simulink model "MX64"  (R2018a)
settings: Solver=VariableStepAuto  StartTime=0.0  StopTime=10.0  MaxStep=2e-04  RelTol=1e-5
values from neighbouring files (symbols this model uses):
  MX106_Te = 1/1000    (= 0.001)    [MX106_init.m]
  MX64_amplifier = MX64_supply_voltage/1024    (= 0.014453125)    [MX64_init.m]
  MX64_inductor = 6.37e-6    (= 6.37e-06)    [MX64_init.m]
  MX64_init_position = 0    [MX64_init.m]
  MX64_Kc = 8e-1    (= 0.8)    [MX64_init.m]
  MX64_Kd = 1/8    (= 0.125)    [MX64_init.m]
  MX64_Ki = 1/1024    (= 0.0009765625)    [MX64_init.m]
  MX64_Kp = 1/8    (= 0.125)    [MX64_init.m]
  MX64_Kv = 9.926e-3    (= 0.009926)    [MX64_init.m]
  MX64_max_speed = 63 * MX64_reduction / 60 * 2 * pi    (= 1319.46891451)    [MX64_init.m]
  MX64_position_gain = 4096 / 2 / pi    (= 651.898646904)    [MX64_init.m]
  MX64_position_offset = pi    (= 3.14159265359)    [MX64_init.m]
  MX64_reduction = 200    [MX64_init.m]
  MX64_stall_current = 5.2    [MX64_init.m]
  MX64_stall_torque = 6.0 / MX64_reduction    (= 0.03)    [MX64_init.m]
  MX64_Te = 1/1000    (= 0.001)    [MX64_init.m]
undefined symbols (not defined in the file or in its folder): MX64_resistor, MX64_speed_gain
libraries: simulink x7, simulink_extras x1
settings Model: Creator=matt  LastModifiedBy=matt

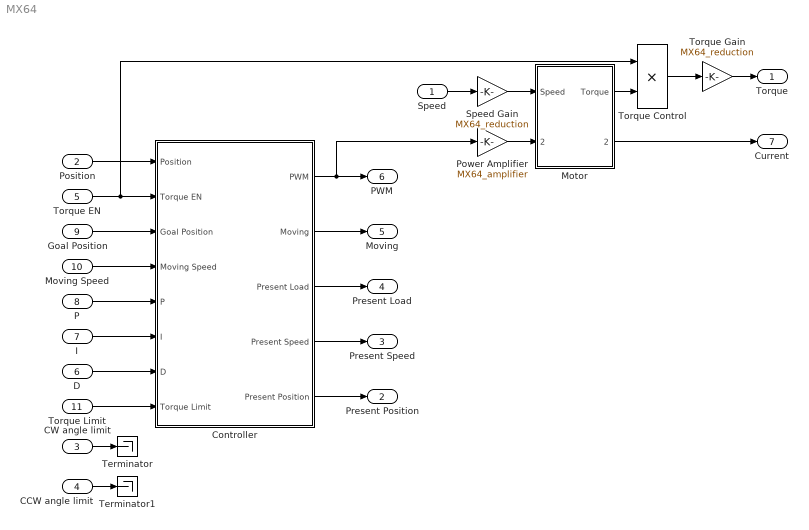
== system MX64 ==
  Speed : Inport
  Position : Inport  Port=2
  CW angle limit : Inport  Port=3  OutDataTypeStr=int16
  CCW angle limit : Inport  Port=4  OutDataTypeStr=int16
  Torque EN : Inport  Port=5  OutDataTypeStr=boolean
  D : Inport  Port=6  OutDataTypeStr=uint8
  I : Inport  Port=7  OutDataTypeStr=uint8
  P : Inport  Port=8  OutDataTypeStr=uint8
  Goal Position : Inport  Port=9
  Moving Speed : Inport  Port=10  OutDataTypeStr=int16
  Torque Limit : Inport  Port=11  OutDataTypeStr=int16
  Controller : Subsystem
  Motor : Subsystem
  Power Amplifier : Gain  Gain=MX64_amplifier  OutDataTypeStr=double
  Speed Gain : Gain  Gain=MX64_reduction
  Terminator : Terminator
  Terminator1 : Terminator
  Torque Control : Product
  Torque Gain : Gain  Gain=MX64_reduction
  Torque : Outport
  Present Position : Outport  Port=2
  Present Speed : Outport  Port=3
  Present Load : Outport  Port=4
  Moving : Outport  Port=5
  PWM : Outport  Port=6
  Current : Outport  Port=7
  wires:
  Controller/5(Present Position) -> Present Position/1
  Controller/3(Present Load) -> Present Load/1
  CW angle limit/1 -> Terminator/1
  Goal Position/1 -> Controller/3(Goal Position)
  Torque Limit/1 -> Controller/8(Torque Limit)
  P/1 -> Controller/5(P)
  Moving Speed/1 -> Controller/4(Moving Speed)
  Torque Control/1 -> Torque Gain/1
  CCW angle limit/1 -> Terminator1/1
  Motor/1(Torque) -> Torque Control/2
  I/1 -> Controller/6(I)
  Torque EN/1 -> Controller/2(Torque EN), Torque Control/1
  Controller/2(Moving) -> Moving/1
  Position/1 -> Controller/1(Position)
  Power Amplifier/1 -> Motor/2(Voltage)
  D/1 -> Controller/7(D)
  Speed/1 -> Speed Gain/1
  Controller/4(Present Speed) -> Present Speed/1
  Controller/1(PWM) -> Power Amplifier/1, PWM/1
  Torque Gain/1 -> Torque/1
  Motor/2(Current) -> Current/1
  Speed Gain/1 -> Motor/1(Speed)

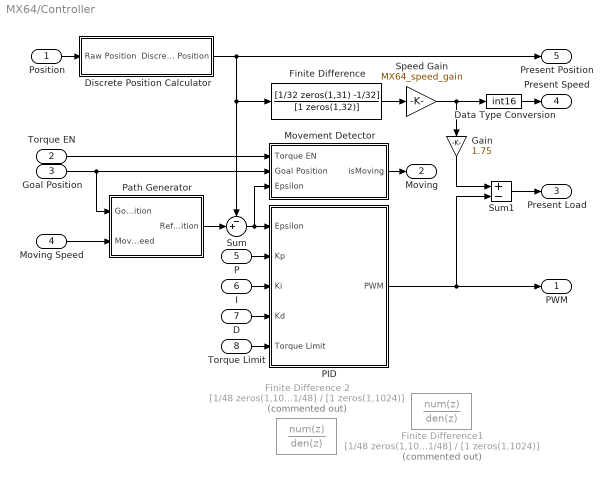
== system MX64/Controller ==
  Position : Inport
  Torque EN : Inport  Port=2
  Goal Position : Inport  Port=3  OutDataTypeStr=int16
  Moving Speed : Inport  Port=4
  P : Inport  Port=5
  I : Inport  Port=6
  D : Inport  Port=7
  Torque Limit : Inport  Port=8
  Data Type Conversion : DataTypeConversion  OutDataTypeStr=int16
  Discrete Position Calculator : Subsystem
  Finite Difference : DiscreteTransferFcn  Numerator=[1/32 zeros(1,31) -1/32]  Denominator=[1 zeros(1,32)]  InitialStates=(MX64_init_position + MX64_position_offset) * MX64_position_gain
  Finite Difference 2 : DiscreteTransferFcn  Commented=on  Numerator=[1/48 zeros(1,1023) -1/48]  Denominator=[1 zeros(1,1024)]  InitialStates=(MX64_init_position + MX64_position_offset) * MX64_position_gain  a0EqualsOne=on
  Finite Difference1 : DiscreteTransferFcn  Commented=on  Numerator=[1/48 zeros(1,1023) -1/48]  Denominator=[1 zeros(1,1024)]  InitialStates=(MX64_init_position + MX64_position_offset) * MX64_position_gain
  Gain : Gain  Gain=1.75  OutDataTypeStr=int16
  Movement Detector : Subsystem
  PID : Subsystem
  Path Generator : Subsystem
  Speed Gain : Gain  Gain=MX64_speed_gain  OutDataTypeStr=double
  Sum : Sum  Inputs=-+|  AccumDataTypeStr=double  OutMin=-4096  OutMax=4096  OutDataTypeStr=double  SaturateOnIntegerOverflow=on
  Sum1 : Sum  Inputs=+-
  PWM : Outport
  Moving : Outport  Port=2
  Present Load : Outport  Port=3
  Present Speed : Outport  Port=4
  Present Position : Outport  Port=5
  wires:
  Movement Detector/1(isMoving) -> Moving/1
  Torque EN/1 -> Movement Detector/1(Torque EN)
  Path Generator/1(Ref Position) -> Sum/2
  Moving Speed/1 -> Path Generator/2(Moving Speed)
  Gain/1 -> Sum1/1
  Sum1/1 -> Present Load/1
  P/1 -> PID/2(Kp)
  I/1 -> PID/3(Ki)
  D/1 -> PID/4(Kd)
  Torque Limit/1 -> PID/5(Torque Limit)
  Data Type Conversion/1 -> Present Speed/1
  Position/1 -> Discrete Position Calculator/1(Raw Position)
  Discrete Position Calculator/1(Discrete Position) -> Finite Difference/1, Sum/1, Present Position/1
  Speed Gain/1 -> Data Type Conversion/1, Gain/1
  PID/1(PWM) -> PWM/1, Sum1/2
  Sum/1 -> PID/1(Epsilon), Movement Detector/3(Epsilon)
  Finite Difference/1 -> Speed Gain/1
  Goal Position/1 -> Path Generator/1(Goal Position), Movement Detector/2(Goal Position)

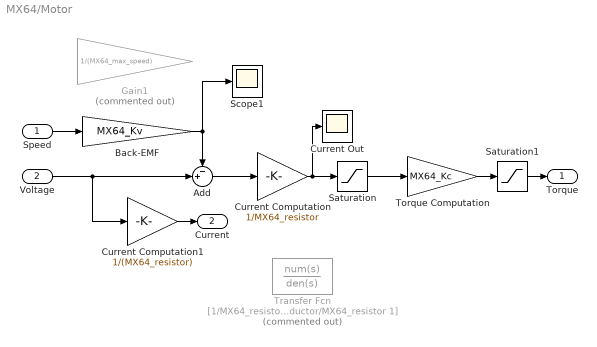
== system MX64/Motor ==
  Speed : Inport
  Voltage : Inport  Port=2
  Add : Sum  Inputs=-+|
  Back-EMF : Gain  Gain=MX64_Kv
  Current Computation : Gain  Gain=1/MX64_resistor
  Current Computation1 : Gain  Gain=1/(MX64_resistor)
  Current Out : Scope
  Gain1 : Gain  Commented=on  Gain=1/(MX64_max_speed)
  Saturation : Saturate  UpperLimit=MX64_stall_current / MX64_reduction  LowerLimit=-MX64_stall_current / MX64_reduction
  Saturation1 : Saturate  UpperLimit=MX64_stall_torque  LowerLimit=-MX64_stall_torque
  Scope1 : Scope
  Torque Computation : Gain  Gain=MX64_Kc
  Transfer Fcn : TransferFcn  Commented=on  Numerator=[1/MX64_resistor]  Denominator=[MX64_inductor/MX64_resistor 1]
  Torque : Outport
  Current : Outport  Port=2
  wires:
  Voltage/1 -> Add/2, Current Computation1/1
  Back-EMF/1 -> Scope1/1, Add/1
  Torque Computation/1 -> Saturation1/1
  Saturation/1 -> Torque Computation/1
  Saturation1/1 -> Torque/1
  Add/1 -> Current Computation/1
  Current Computation1/1 -> Current/1
  Speed/1 -> Back-EMF/1
  Current Computation/1 -> Current Out/1, Saturation/1

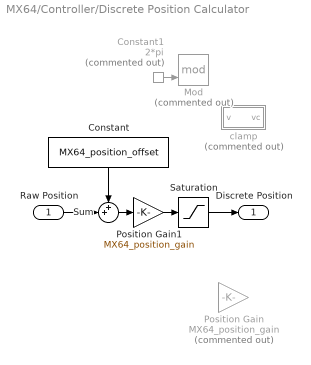
== system MX64/Controller/Discrete Position Calculator ==
  Raw Position : Inport
  Constant : Constant  Value=MX64_position_offset  SampleTime=-1
  Constant1 : Constant  Commented=on  Value=2*pi
  Mod : Math  Commented=on  Operator=mod  SaturateOnIntegerOverflow=on
  Position Gain : Gain  Commented=on  Gain=MX64_position_gain  OutMin=0  OutMax=4095  OutDataTypeStr=int16  SaturateOnIntegerOverflow=on
  Position Gain1 : Gain  Gain=MX64_position_gain  OutMin=0  OutMax=4095  OutDataTypeStr=int16  SampleTime=MX64_Te  SaturateOnIntegerOverflow=on
  Saturation : Saturate  UpperLimit=4095  LowerLimit=0  ZeroCross=off
  Sum : Sum  Inputs=++|
  clamp : Subsystem  Commented=on
  Discrete Position : Outport
  wires:
  Position Gain1/1 -> Saturation/1
  Constant/1 -> Sum/1
  Raw Position/1 -> Sum/2
  Sum/1 -> Position Gain1/1
  ? -> Mod/1
  Constant1/1 -> Mod/2
  Saturation/1 -> Discrete Position/1

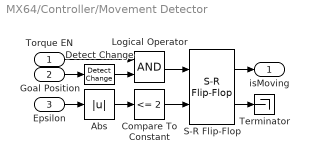
== system MX64/Controller/Movement Detector ==
  Torque EN : Inport
  Goal Position : Inport  Port=2
  Epsilon : Inport  Port=3
  Abs : Abs  ZeroCross=off
  Compare To Constant : simulink/Logic and Bit Operations/Compare To Constant  relop=<=  const=2  OutDataTypeStr=boolean  ZeroCross=off
  Detect Change : simulink/Logic and Bit Operations/Detect Change  vinit=0  OutDataTypeStr=boolean
  Logical Operator : Logic  AllPortsSameDT=off  OutDataTypeStr=boolean
  S-R Flip-Flop : simulink_extras/Flip Flops/S-R Flip-Flop  initial_condition=0
  Terminator : Terminator
  isMoving : Outport
  wires:
  Compare To Constant/1 -> S-R Flip-Flop/2
  Abs/1 -> Compare To Constant/1
  Goal Position/1 -> Detect Change/1
  Detect Change/1 -> Logical Operator/2
  S-R Flip-Flop/2 -> Terminator/1
  Logical Operator/1 -> S-R Flip-Flop/1
  Epsilon/1 -> Abs/1
  S-R Flip-Flop/1 -> isMoving/1
  Torque EN/1 -> Logical Operator/1

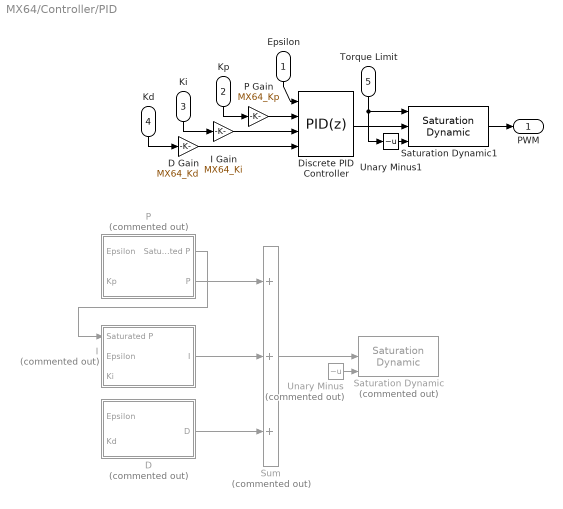
== system MX64/Controller/PID ==
  Epsilon : Inport
  Kp : Inport  Port=2
  Ki : Inport  Port=3
  Kd : Inport  Port=4
  Torque Limit : Inport  Port=5
  D : Subsystem  Commented=on
  D Gain : Gain  Gain=MX64_Kd  OutDataTypeStr=double
  Discrete PID Controller : simulink/Continuous/PID Controller  Controller=PID  TimeDomain=Discrete-time  SampleTime=-1  IntegratorMethod=Forward Euler  FilterMethod=Forward Euler  Form=Parallel  UseFilter=off  ControllerParametersSource=external  P=1  I=1  D=0  N=100  InitialConditionSource=internal  InitialConditionForIntegrator=0  InitialConditionForFilter=0  ExternalReset=none  LimitOutput=off  UpperSaturationLimit=inf  LowerSaturationLimit=-inf  LinearizeAsGain=off  AntiWindupMode=none  Kb=1  TrackingMode=off  Kt=1  PParamMin=[]  PParamMax=[]  IParamMin=[]  IParamMax=[]  DParamMin=[]  DParamMax=[]  NParamMin=[]  NParamMax=[]  KbParamMin=[]  KbParamMax=[]  KtParamMin=[]  KtParamMax=[]  POutMin=[]  POutMax=[]  IOutMin=[]  IOutMax=[]  DOutMin=[]  DOutMax=[]  NOutMin=[]  NOutMax=[]  KbOutMin=[]  KbOutMax=[]  KtOutMin=[]  KtOutMax=[]  IntegratorOutMin=[]  IntegratorOutMax=[]  FilterOutMin=[]  FilterOutMax=[]  SumOutMin=[]  SumOutMax=[]  SumOutDataTypeStr=int16  SumI1OutMin=[]  SumI1OutMax=[]  SumI2OutMin=[]  SumI2OutMax=[]  SumI3OutMin=[]  SumI3OutMax=[]  SumDOutMin=[]  SumDOutMax=[]  SaturationOutMin=[]  SaturationOutMax=[]  IntegratorContinuousStateAttributes=''  IntegratorStateMustResolveToSignalObject=off  IntegratorRTWStateStorageClass=Auto  FilterContinuousStateAttributes=''  FilterStateMustResolveToSignalObject=off  FilterRTWStateStorageClass=Auto  DifferentiatorICPrevScaledInput=0  DifferentiatorOutMin=[]  DifferentiatorOutMax=[]  FilterDiffOutCoefMin=[]  FilterDiffOutCoefMax=[]  SumDenOutMin=[]  SumDenOutMax=[]  SumNumOutMin=[]  SumNumOutMax=[]  ReciprocalOutMin=[]  ReciprocalOutMax=[]  DivideOutMin=[]  DivideOutMax=[]  TunerSelectOption=Transfer Function Based (PID Tuner App)
  I : Subsystem  Commented=on
  I Gain : Gain  Gain=MX64_Ki  OutDataTypeStr=double
  P : Subsystem  Commented=on
  P Gain : Gain  Gain=MX64_Kp  OutDataTypeStr=double
  Saturation Dynamic : simulink/Discontinuities/Saturation Dynamic  Commented=on  OutMin=[]  OutMax=[]  OutDataTypeStr=Inherit: Same as second input  OutDataType=fixdt(1, 16)  OutScaling=2^-10  DoSatur=off
  Saturation Dynamic1 : simulink/Discontinuities/Saturation Dynamic  OutMin=[]  OutMax=[]  OutDataTypeStr=Inherit: Same as second input  OutDataType=fixdt(1, 16)  OutScaling=2^-10  DoSatur=off
  Sum : Sum  Commented=on  Inputs=3  OutDataTypeStr=int16  SaturateOnIntegerOverflow=on
  Unary Minus : UnaryMinus  Commented=on
  Unary Minus1 : UnaryMinus
  PWM : Outport
  wires:
  Unary Minus/1 -> Saturation Dynamic/3
  Sum/1 -> Saturation Dynamic/2
  Epsilon/1 -> Discrete PID Controller/1
  Kp/1 -> P Gain/1
  P/2(P) -> Sum/1
  P/1(Saturated P) -> I/1(Saturated P)
  Ki/1 -> I Gain/1
  I/1(I) -> Sum/2
  D/1(D) -> Sum/3
  P Gain/1 -> Discrete PID Controller/2
  I Gain/1 -> Discrete PID Controller/3
  D Gain/1 -> Discrete PID Controller/4
  Discrete PID Controller/1 -> Saturation Dynamic1/2
  Unary Minus1/1 -> Saturation Dynamic1/3
  Saturation Dynamic1/1 -> PWM/1
  Torque Limit/1 -> Saturation Dynamic1/1, Unary Minus1/1
  Kd/1 -> D Gain/1

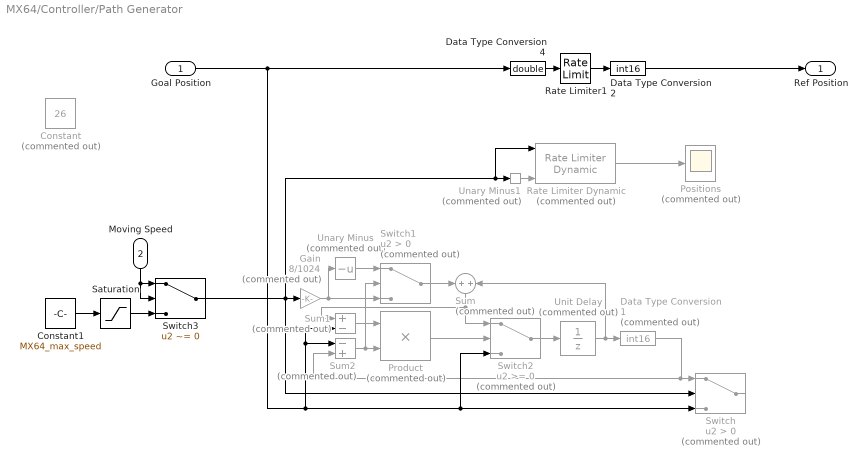
== system MX64/Controller/Path Generator ==
  Goal Position : Inport
  Moving Speed : Inport  Port=2
  Constant : Constant  Commented=on  Value=26
  Constant1 : Constant  Value=MX64_max_speed
  Data Type Conversion1 : DataTypeConversion  Commented=on  OutDataTypeStr=int16
  Data Type Conversion2 : DataTypeConversion  OutDataTypeStr=int16
  Data Type Conversion4 : DataTypeConversion  OutDataTypeStr=double
  Gain : Gain  Commented=on  Gain=8/1024  ParamDataTypeStr=double
  Positions : Scope  Commented=on  NumInputPorts=3
  Product : Product  Commented=on
  Rate Limiter Dynamic : simulink/Discontinuities/Rate Limiter Dynamic  Commented=on
      settings: SourceProductName=Simulink
  Rate Limiter1 : RateLimiter  RisingSlewLimit=MX64_max_speed  FallingSlewLimit=-MX64_max_speed  SampleTimeMode=inherited  InitialCondition=(MX64_init_position + MX64_position_offset) * MX64_position_gain
  Saturation : Saturate  UpperLimit=1023  LowerLimit=0  ZeroCross=off
  Sum : Sum  Commented=on  Inputs=+|+
  Sum1 : Sum  Commented=on  Inputs=+-
  Sum2 : Sum  Commented=on  Inputs=-+
  Switch : Switch  Commented=on  Criteria=u2 > Threshold  ZeroCross=off
  Switch1 : Switch  Commented=on  Criteria=u2 > Threshold  ZeroCross=off
  Switch2 : Switch  Commented=on  ZeroCross=off
  Switch3 : Switch  Criteria=u2 ~= 0  ZeroCross=off
  Unary Minus : UnaryMinus  Commented=on
  Unary Minus1 : UnaryMinus  Commented=on
  Unit Delay : UnitDelay  Commented=on  InitialCondition=(MX64_init_position+MX64_position_offset) * MX64_position_gain  SampleTime=-1
  Ref Position : Outport
  wires:
  Sum/1 -> Switch2/1, Sum1/1
  Switch2/1 -> Unit Delay/1
  Unit Delay/1 -> Sum/2, Data Type Conversion1/1
  Switch1/1 -> Sum/1
  Data Type Conversion1/1 -> Sum2/2, Switch/1
  Sum1/1 -> Product/1
  Sum2/1 -> Switch1/2, Product/2
  Product/1 -> Switch2/2
  Unary Minus/1 -> Switch1/1
  Gain/1 -> Switch1/3, Unary Minus/1
  Moving Speed/1 -> Switch3/2, Switch3/1
  Constant1/1 -> Saturation/1
  Saturation/1 -> Switch3/3
  Unary Minus1/1 -> Rate Limiter Dynamic/3
  Data Type Conversion2/1 -> Ref Position/1
  Data Type Conversion4/1 -> Rate Limiter1/1
  Rate Limiter1/1 -> Data Type Conversion2/1
  Switch3/1 -> Switch/2, Gain/1, Rate Limiter Dynamic/1, Unary Minus1/1
  Rate Limiter Dynamic/1 -> Positions/2
  Goal Position/1 -> Data Type Conversion4/1, Switch2/3, Switch/3, Sum2/1, Sum1/2

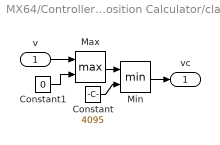
== system MX64/Controller/Discrete Position Calculator/clamp ==
  v : Inport
  Constant : Constant  Value=4095
  Constant1 : Constant  Value=0
  Max : MinMax  Function=max  Inputs=2
  Min : MinMax  Inputs=2
  vc : Outport
  wires:
  Constant1/1 -> Max/2
  Min/1 -> vc/1
  v/1 -> Max/1
  Max/1 -> Min/1
  Constant/1 -> Min/2

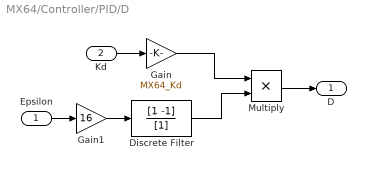
== system MX64/Controller/PID/D ==
  Epsilon : Inport
  Kd : Inport  Port=2
  Discrete Filter : DiscreteFilter  Numerator=[1 -1]  Denominator=[1]  a0EqualsOne=on
  Gain : Gain  Gain=MX64_Kd  OutDataTypeStr=double
  Gain1 : Gain  Gain=16
  Multiply : Product
  D : Outport
  wires:
  Discrete Filter/1 -> Multiply/2
  Kd/1 -> Gain/1
  Epsilon/1 -> Gain1/1
  Gain/1 -> Multiply/1
  Multiply/1 -> D/1
  Gain1/1 -> Discrete Filter/1

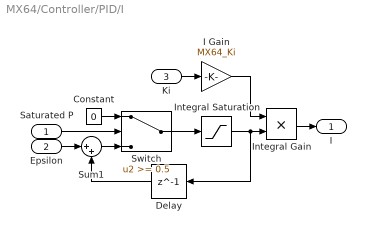
== system MX64/Controller/PID/I ==
  Saturated P : Inport
  Epsilon : Inport  Port=2
  Ki : Inport  Port=3
  Constant : Constant  Value=0
  Delay : Delay  DelayLength=1  SampleTime=MX106_Te
  I Gain : Gain  Gain=MX64_Ki  OutDataTypeStr=double
  Integral Gain : Product
  Integral Saturation : Saturate  UpperLimit=30690  LowerLimit=-30690  ZeroCross=off
  Sum1 : Sum  Inputs=|++
  Switch : Switch  Threshold=0.5  ZeroCross=off
  I : Outport
  wires:
  Saturated P/1 -> Switch/2
  I Gain/1 -> Integral Gain/1
  Ki/1 -> I Gain/1
  Constant/1 -> Switch/1
  Switch/1 -> Integral Saturation/1
  Epsilon/1 -> Sum1/1
  Integral Gain/1 -> I/1
  Delay/1 -> Sum1/2
  Sum1/1 -> Switch/3
  Integral Saturation/1 -> Delay/1, Integral Gain/2

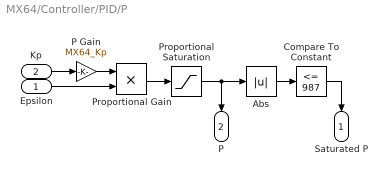
== system MX64/Controller/PID/P ==
  Epsilon : Inport
  Kp : Inport  Port=2
  Abs : Abs  ZeroCross=off
  Compare To Constant : simulink/Logic and Bit Operations/Compare To Constant  relop=<=  const=987  OutDataTypeStr=boolean  ZeroCross=off
  P Gain : Gain  Gain=MX64_Kp  OutDataTypeStr=double
  Proportional Gain : Product
  Proportional Saturation : Saturate  UpperLimit=987  LowerLimit=-987  ZeroCross=off
  Saturated P : Outport
  P : Outport  Port=2
  wires:
  P Gain/1 -> Proportional Gain/1
  Abs/1 -> Compare To Constant/1
  Epsilon/1 -> Proportional Gain/2
  Proportional Saturation/1 -> Abs/1, P/1
  Compare To Constant/1 -> Saturated P/1
  Proportional Gain/1 -> Proportional Saturation/1
  Kp/1 -> P Gain/1
